simulink model "Project3_System_partA"  (R2018b)
settings: Solver=VariableStepAuto  StartTime=0.0  StopTime=10  FixedStep=.001  MaxStep=.001  RelTol=1e-6  EnableMultiTasking=on
values from neighbouring files (symbols this model uses):
  Kd = 700    [SimRun.m]
  Kp = 1000    [SimRun.m]
  n = link.inertia*(iwdot) + cross(iw, link.inertia*iw)    [newtonEuler.m]
  points = points3D    [SimRun.m]
  transPercent = 0.025    [SimRun.m]
(part 4 of 4)

== matlab function Project3_System_partA/MATLAB Function ==
  data: theta input; theta_ddot input; torque output; theta_dot input
function torque = newton_euler( theta, theta_ddot, theta_dot )
%#codegen
coder.extrinsic('evalin');
coder.extrinsic('newtonEuler');

persistent linkList boundry_conditions;

if isempty(linkList)
    linkList = evalin('base','linkList');
    boundry_conditions.base_angular_velocity = [0;0;0];
    boundry_conditions.base_angular_acceleration = [0;0;0];
    boundry_conditions.base_linear_acceleration = [0;0;9.8];
    boundry_conditions.distal_force = [0;0;0];
    boundry_conditions.distal_torque = [0;0;0];
end

theta(2) = theta(2)-pi/2; % put in DH frame
torque = zeros(6,1);
torque = newtonEuler(linkList,theta,theta_dot,theta_ddot,boundry_conditions);


end

== matlab function Project3_System_partA/ABB Arm Dynamics/Laser Tracking ==
  data: theta input; pose output
function pose = laserTracker(theta)
%#codegen
coder.extrinsic('evalin');
persistent Sim_Exact;

if isempty(Sim_Exact)
    Sim_Exact = evalin('base','Sim_Exact');
end


th1 = theta(1);
th2 = theta(2);
th3 = theta(3);
th4 = theta(4);
th5 = theta(5);
th6 = theta(6);


if(Sim_Exact)
    pose = [ sin(th6)*(cos(th4)*sin(th1) + sin(th4)*(cos(th1)*sin(th2)*sin(th3) - cos(th1)*cos(th2)*cos(th3))) + cos(th6)*(cos(th5)*(sin(th1)*sin(th4) - cos(th4)*(cos(th1)*sin(th2)*sin(th3) - cos(th1)*cos(th2)*cos(th3))) - sin(th5)*(cos(th1)*cos(th2)*sin(th3) + cos(th1)*cos(th3)*sin(th2))), cos(th6)*(cos(th4)*sin(th1) + sin(th4)*(cos(th1)*sin(th2)*sin(th3) - cos(th1)*cos(th2)*cos(th3))) - sin(th6)*(cos(th5)*(sin(th1)*sin(th4) - cos(th4)*(cos(th1)*sin(th2)*sin(th3) - cos(th1)*cos(th2)*cos(th3))) - sin(th5)*(cos(th1)*cos(th2)*sin(th3) + cos(th1)*cos(th3)*sin(th2))), - sin(th5)*(sin(th1)*sin(th4) - cos(th4)*(cos(th1)*sin(th2)*sin(th3) - cos(th1)*cos(th2)*cos(th3))) - cos(th5)*(cos(th1)*cos(th2)*sin(th3) + cos(th1)*cos(th3)*sin(th2)), (27*cos(th1)*cos(th2))/100 - (9*sin(th5)*(sin(th1)*sin(th4) - cos(th4)*(cos(th1)*sin(th2)*sin(th3) - cos(th1)*cos(th2)*cos(th3))))/125 - (9*cos(th5)*(cos(th1)*cos(th2)*sin(th3) + cos(th1)*cos(th3)*sin(th2)))/125 - (7*cos(th1)*sin(th2)*sin(th3))/100 + (7*cos(th1)*cos(th2)*cos(th3))/100 - (151*cos(th1)*cos(th2)*sin(th3))/500 - (151*cos(th1)*cos(th3)*sin(th2))/500;
        - sin(th6)*(cos(th1)*cos(th4) - sin(th4)*(sin(th1)*sin(th2)*sin(th3) - cos(th2)*cos(th3)*sin(th1))) - cos(th6)*(cos(th5)*(cos(th1)*sin(th4) + cos(th4)*(sin(th1)*sin(th2)*sin(th3) - cos(th2)*cos(th3)*sin(th1))) + sin(th5)*(cos(th2)*sin(th1)*sin(th3) + cos(th3)*sin(th1)*sin(th2))), sin(th6)*(cos(th5)*(cos(th1)*sin(th4) + cos(th4)*(sin(th1)*sin(th2)*sin(th3) - cos(th2)*cos(th3)*sin(th1))) + sin(th5)*(cos(th2)*sin(th1)*sin(th3) + cos(th3)*sin(th1)*sin(th2))) - cos(th6)*(cos(th1)*cos(th4) - sin(th4)*(sin(th1)*sin(th2)*sin(th3) - cos(th2)*cos(th3)*sin(th1))), sin(th5)*(cos(th1)*sin(th4) + cos(th4)*(sin(th1)*sin(th2)*sin(th3) - cos(th2)*cos(th3)*sin(th1))) - cos(th5)*(cos(th2)*sin(th1)*sin(th3) + cos(th3)*sin(th1)*sin(th2)), (27*cos(th2)*sin(th1))/100 + (9*sin(th5)*(cos(th1)*sin(th4) + cos(th4)*(sin(th1)*sin(th2)*sin(th3) - cos(th2)*cos(th3)*sin(th1))))/125 - (9*cos(th5)*(cos(th2)*sin(th1)*sin(th3) + cos(th3)*sin(th1)*sin(th2)))/125 - (151*cos(th2)*sin(th1)*sin(th3))/500 - (151*cos(th3)*sin(th1)*sin(th2))/500 - (7*sin(th1)*sin(th2)*sin(th3))/100 + (7*cos(th2)*cos(th3)*sin(th1))/100;
        sin(th4)*sin(th6)*(cos(th2)*sin(th3) + cos(th3)*sin(th2)) - cos(th6)*(sin(th5)*(cos(th2)*cos(th3) - sin(th2)*sin(th3)) + cos(th4)*cos(th5)*(cos(th2)*sin(th3) + cos(th3)*sin(th2))), sin(th6)*(sin(th5)*(cos(th2)*cos(th3) - sin(th2)*sin(th3)) + cos(th4)*cos(th5)*(cos(th2)*sin(th3) + cos(th3)*sin(th2))) + cos(th6)*sin(th4)*(cos(th2)*sin(th3) + cos(th3)*sin(th2)), cos(th4)*sin(th5)*(cos(th2)*sin(th3) + cos(th3)*sin(th2)) - cos(th5)*(cos(th2)*cos(th3) - sin(th2)*sin(th3)), (151*sin(th2)*sin(th3))/500 - (151*cos(th2)*cos(th3))/500 - (7*cos(th2)*sin(th3))/100 - (7*cos(th3)*sin(th2))/100 - (27*sin(th2))/100 - (9*cos(th5)*(cos(th2)*cos(th3) - sin(th2)*sin(th3)))/125 + (9*cos(th4)*sin(th5)*(cos(th2)*sin(th3) + cos(th3)*sin(th2)))/125 + 29/100;
        0, 0, 0, 1];
else
    
    pose = [ sin(th6)*(cos(th4)*sin(th1) + sin(th4)*(cos(th1)*sin(th2)*sin(th3) - cos(th1)*cos(th2)*cos(th3))) + cos(th6)*(cos(th5)*(sin(th1)*sin(th4) - cos(th4)*(cos(th1)*sin(th2)*sin(th3) - cos(th1)*cos(th2)*cos(th3))) - sin(th5)*(cos(th1)*cos(th2)*sin(th3) + cos(th1)*cos(th3)*sin(th2))), cos(th6)*(cos(th4)*sin(th1) + sin(th4)*(cos(th1)*sin(th2)*sin(th3) - cos(th1)*cos(th2)*cos(th3))) - sin(th6)*(cos(th5)*(sin(th1)*sin(th4) - cos(th4)*(cos(th1)*sin(th2)*sin(th3) - cos(th1)*cos(th2)*cos(th3))) - sin(th5)*(cos(th1)*cos(th2)*sin(th3) + cos(th1)*cos(th3)*sin(th2))), - sin(th5)*(sin(th1)*sin(th4) - cos(th4)*(cos(th1)*sin(th2)*sin(th3) - cos(th1)*cos(th2)*cos(th3))) - cos(th5)*(cos(th1)*cos(th2)*sin(th3) + cos(th1)*cos(th3)*sin(th2)), (151838081588107*cos(th1)*cos(th2))/562949953421312 - (123928564092639*sin(th1))/72057594037927936 - (7184037743251309*cos(th1))/36893488147419103232 - (7330531551818703*cos(th4)*sin(th1))/36893488147419103232 - (5489399374888815*sin(th1)*sin(th4))/9223372036854775808 + (970893499285375*cos(th5)*(sin(th1)*sin(th4) - cos(th4)*(cos(th1)*sin(th2)*sin(th3) - cos(th1)*cos(th2)*cos(th3))))/9223372036854775808 - (5192391675427195*sin(th5)*(sin(th1)*sin(th4) - cos(th4)*(cos(th1)*sin(th2)*sin(th3) - cos(th1)*cos(th2)*cos(th3))))/72057594037927936 + (1663072680156839*sin(th6)*(cos(th4)*sin(th1) + sin(th4)*(cos(th1)*sin(th2)*sin(th3) - cos(th1)*cos(th2)*cos(th3))))/2305843009213693952 + (1663072680156839*cos(th6)*(cos(th5)*(sin(th1)*sin(th4) - cos(th4)*(cos(th1)*sin(th2)*sin(th3) - cos(th1)*cos(th2)*cos(th3))) - sin(th5)*(cos(th1)*cos(th2)*sin(th3) + cos(th1)*cos(th3)*sin(th2))))/2305843009213693952 + (5489399374888815*cos(th4)*(cos(th1)*sin(th2)*sin(th3) - cos(th1)*cos(th2)*cos(th3)))/9223372036854775808 - (5192391675427195*cos(th5)*(cos(th1)*cos(th2)*sin(th3) + cos(th1)*cos(th3)*sin(th2)))/72057594037927936 - (7330531551818703*sin(th4)*(cos(th1)*sin(th2)*sin(th3) - cos(th1)*cos(th2)*cos(th3)))/36893488147419103232 - (970893499285375*sin(th5)*(cos(th1)*cos(th2)*sin(th3) + cos(th1)*cos(th3)*sin(th2)))/9223372036854775808 - (1259578569946919*cos(th1)*sin(th2)*sin(th3))/18014398509481984 + (1259578569946919*cos(th1)*cos(th2)*cos(th3))/18014398509481984 - (5430591396830085*cos(th1)*cos(th2)*sin(th3))/18014398509481984 - (5430591396830085*cos(th1)*cos(th3)*sin(th2))/18014398509481984;
        - sin(th6)*(cos(th1)*cos(th4) - sin(th4)*(sin(th1)*sin(th2)*sin(th3) - cos(th2)*cos(th3)*sin(th1))) - cos(th6)*(cos(th5)*(cos(th1)*sin(th4) + cos(th4)*(sin(th1)*sin(th2)*sin(th3) - cos(th2)*cos(th3)*sin(th1))) + sin(th5)*(cos(th2)*sin(th1)*sin(th3) + cos(th3)*sin(th1)*sin(th2))), sin(th6)*(cos(th5)*(cos(th1)*sin(th4) + cos(th4)*(sin(th1)*sin(th2)*sin(th3) - cos(th2)*cos(th3)*sin(th1))) + sin(th5)*(cos(th2)*sin(th1)*sin(th3) + cos(th3)*sin(th1)*sin(th2))) - cos(th6)*(cos(th1)*cos(th4) - sin(th4)*(sin(th1)*sin(th2)*sin(th3) - cos(th2)*cos(th3)*sin(th1))), sin(th5)*(cos(th1)*sin(th4) + cos(th4)*(sin(th1)*sin(th2)*sin(th3) - cos(th2)*cos(th3)*sin(th1))) - cos(th5)*(cos(th2)*sin(th1)*sin(th3) + cos(th3)*sin(th1)*sin(th2)), (123928564092639*cos(th1))/72057594037927936 - (7184037743251309*sin(th1))/36893488147419103232 + (7330531551818703*cos(th1)*cos(th4))/36893488147419103232 + (151838081588107*cos(th2)*sin(th1))/562949953421312 + (5489399374888815*cos(th1)*sin(th4))/9223372036854775808 - (970893499285375*cos(th5)*(cos(th1)*sin(th4) + cos(th4)*(sin(th1)*sin(th2)*sin(th3) - cos(th2)*cos(th3)*sin(th1))))/9223372036854775808 + (5192391675427195*sin(th5)*(cos(th1)*sin(th4) + cos(th4)*(sin(th1)*sin(th2)*sin(th3) - cos(th2)*cos(th3)*sin(th1))))/72057594037927936 - (1663072680156839*sin(th6)*(cos(th1)*cos(th4) - sin(th4)*(sin(th1)*sin(th2)*sin(th3) - cos(th2)*cos(th3)*sin(th1))))/2305843009213693952 + (5489399374888815*cos(th4)*(sin(th1)*sin(th2)*sin(th3) - cos(th2)*cos(th3)*sin(th1)))/9223372036854775808 - (5192391675427195*cos(th5)*(cos(th2)*sin(th1)*sin(th3) + cos(th3)*sin(th1)*sin(th2)))/72057594037927936 - (1663072680156839*cos(th6)*(cos(th5)*(cos(th1)*sin(th4) + cos(th4)*(sin(th1)*sin(th2)*sin(th3) - cos(th2)*cos(th3)*sin(th1))) + sin(th5)*(cos(th2)*sin(th1)*sin(th3) + cos(th3)*sin(th1)*sin(th2))))/2305843009213693952 - (7330531551818703*sin(th4)*(sin(th1)*sin(th2)*sin(th3) - cos(th2)*cos(th3)*sin(th1)))/36893488147419103232 - (970893499285375*sin(th5)*(cos(th2)*sin(th1)*sin(th3) + cos(th3)*sin(th1)*sin(th2)))/9223372036854775808 - (5430591396830085*cos(th2)*sin(th1)*sin(th3))/18014398509481984 - (5430591396830085*cos(th3)*sin(th1)*sin(th2))/18014398509481984 - (1259578569946919*sin(th1)*sin(th2)*sin(th3))/18014398509481984 + (1259578569946919*cos(th2)*cos(th3)*sin(th1))/18014398509481984;
        sin(th4)*sin(th6)*(cos(th2)*sin(th3) + cos(th3)*sin(th2)) - cos(th6)*(sin(th5)*(cos(th2)*cos(th3) - sin(th2)*sin(th3)) + cos(th4)*cos(th5)*(cos(th2)*sin(th3) + cos(th3)*sin(th2))), sin(th6)*(sin(th5)*(cos(th2)*cos(th3) - sin(th2)*sin(th3)) + cos(th4)*cos(th5)*(cos(th2)*sin(th3) + cos(th3)*sin(th2))) + cos(th6)*sin(th4)*(cos(th2)*sin(th3) + cos(th3)*sin(th2)), cos(th4)*sin(th5)*(cos(th2)*sin(th3) + cos(th3)*sin(th2)) - cos(th5)*(cos(th2)*cos(th3) - sin(th2)*sin(th3)), (5430591396830085*sin(th2)*sin(th3))/18014398509481984 - (5430591396830085*cos(th2)*cos(th3))/18014398509481984 - (1259578569946919*cos(th2)*sin(th3))/18014398509481984 - (1259578569946919*cos(th3)*sin(th2))/18014398509481984 - (1663072680156839*cos(th6)*(sin(th5)*(cos(th2)*cos(th3) - sin(th2)*sin(th3)) + cos(th4)*cos(th5)*(cos(th2)*sin(th3) + cos(th3)*sin(th2))))/2305843009213693952 - (151838081588107*sin(th2))/562949953421312 + (5489399374888815*cos(th4)*(cos(th2)*sin(th3) + cos(th3)*sin(th2)))/9223372036854775808 - (5192391675427195*cos(th5)*(cos(th2)*cos(th3) - sin(th2)*sin(th3)))/72057594037927936 - (7330531551818703*sin(th4)*(cos(th2)*sin(th3) + cos(th3)*sin(th2)))/36893488147419103232 - (970893499285375*sin(th5)*(cos(th2)*cos(th3) - sin(th2)*sin(th3)))/9223372036854775808 - (970893499285375*cos(th4)*cos(th5)*(cos(th2)*sin(th3) + cos(th3)*sin(th2)))/9223372036854775808 + (5192391675427195*cos(th4)*sin(th5)*(cos(th2)*sin(th3) + cos(th3)*sin(th2)))/72057594037927936 + (1663072680156839*sin(th4)*sin(th6)*(cos(th2)*sin(th3) + cos(th3)*sin(th2)))/2305843009213693952 + 325695105792877/1125899906842624;
        0, 0, 0, 1];
end

== matlab function Project3_System_partA/MATLAB Function1 ==
  data: t input; theta_des output; points input; n input
function theta_des = abb(t,points,n)
theta_des = zeros(length(t),7);
thetaa = zeros(length(t),7);
th_last=[0;-pi/2;0;0;0;0];
th1=0;
th2=0;
th3=0;
th4=0;
th5=0;
th6=0;
R=zeros(3,3);
x_vec=zeros(3,1);
y_vec=zeros(3,1);
z_vec=zeros(3,1);
% [n,V,p] = affine_fit(points);
z_vec=real(n);

thetaa(1,2:7)=-1*th_last';
thetaa(1,1)=t(1);
diff=points(2,:)-points(1,:);
x_vec=diff'/norm(diff);
y_vec=cpMap(z_vec)*x_vec;
R=[x_vec y_vec z_vec];
[th1,th2,th3,th4,th5,th6,~]=abbInvKine([R points(1,:)';0 0 0 1],th_last);
thetaa(2,2:7)=[th1,th2,th3,th4,th5,th6];
thetaa(2,1)=t(2);
[th1,th2,th3,th4,th5,th6,~]=abbInvKine([R points(1,:)';0 0 0 1],th_last);
thetaa(3,2:7)=[th1,th2,th3,th4,th5,th6];
thetaa(3,1)=t(3);
for i=3:length(t)-2
    diff=points(i-1,:)-points(i-2,:);
    x_vec=diff'/norm(diff);
    y_vec=cpMap(z_vec)*x_vec;
    R=[x_vec y_vec z_vec];
[th1,th2,th3,th4,th5,th6,~]=abbInvKine([R points(i-1,:)';0 0 0 1],thetaa(i,2:7)');
thetaa(i+1,2:7)=[th1,th2,th3,th4,th5,th6];
% for j=2:7
% if thetaa(i+1,j)*thetaa(i,j)' <0
% thetaa(i+1,j)=-1*thetaa(i+1,j);
% end
% end
thetaa(i+1,1)=t(i+1);
thetaa(i+2,2:7)=thetaa(i+1,2:7);
thetaa(i+2,1)=t(i+2);
end
theta_des = thetaa;
end

== matlab function Project3_System_partA/MATLAB Function2 ==
  data: t input double; theta output double; trajectory input double; transPercent input double; theta_dot output double
function [theta,theta_dot] = constAccelInterp(t,trajectory,transPercent)
pTime = trajectory(:,1);
[n,m] = size(trajectory);
thetaa = zeros(1,m-1);
thetaa_dot = zeros(1,m-1);
a = zeros(1,m-1);
for j = 2:n-1
    if j-1==1 && t>=pTime(j-1,1) && t<=(pTime(j-1,1)+transPercent)
        for i = 2:m
            thetaa(1,i-1) = trajectory(j-1,i) +...
                (((trajectory(j,i)-trajectory(j-1,i))*((t-pTime(j-1,1)+transPercent)^2))/(4*transPercent*(pTime(j,1)-pTime(j-1,1))));
            thetaa_dot(1,i-1) = (((trajectory(j,i)-trajectory(j-1,i))*(t-pTime(j-1,1)+transPercent))/(2*transPercent*(pTime(j,1)-pTime(j-1,1))));
            a(1,i-1) = ((trajectory(j,i)-trajectory(j-1,i))/(2*transPercent*(pTime(j,1)-pTime(j-1,1))));
        end
        break;
    elseif j+1==n && t>=(pTime(j+1,1)-transPercent) && t<=pTime(j+1,1)
        for i = 2:m
            thetaa(1,i-1) = trajectory(j+1,i) - ...
                (((trajectory(j+1,i)-trajectory(j,i))*((t-pTime(j+1,1)-transPercent)^2))/(4*transPercent*(pTime(j+1,1)-pTime(j,1))));
            thetaa_dot(1,i-1) = -(((trajectory(j+1,i)-trajectory(j,i))*(t-pTime(j+1,1)-transPercent))/(2*transPercent*(pTime(j+1,1)-pTime(j,1))));
            a(1,i-1) = -((trajectory(j+1,i)-trajectory(j,i))/(2*transPercent*(pTime(j+1,1)-pTime(j,1))));
        end
        break;
    elseif t>=(pTime(j-1,1)+transPercent) && t<=(pTime(j,1)-transPercent)
        for i = 2:m
            thetaa(1,i-1) = trajectory(j,i)-(((pTime(j,1)-t)*(trajectory(j,i)-...
                trajectory(j-1,i)))/(pTime(j,1)-pTime(j-1,1)));
            thetaa_dot(1,i-1) = (trajectory(j,i)-trajectory(j-1,i))/(pTime(j,1)-pTime(j-1,1));
            a(1,i-1) = 0.0;
        end
        break;
    elseif t>=(pTime(j,1)-transPercent) && t<=(pTime(j,1)+transPercent)
        for i = 2:m
            thetaa(1,i-1) = trajectory(j,i) - ...
                (((trajectory(j,i)-trajectory(j-1,i))*((t-pTime(j,1)-transPercent)^2))/(4*transPercent*(pTime(j,1)-pTime(j-1,1)))) +...
                (((trajectory(j+1,i)-trajectory(j,i))*((t-pTime(j,1)+transPercent)^2))/(4*transPercent*(pTime(j+1,1)-pTime(j,1))));
            thetaa_dot(1,i-1) = -(((trajectory(j,i)-trajectory(j-1,i))*(t-pTime(j,1)-transPercent))/(2*transPercent*(pTime(j,1)-pTime(j-1,1)))) +...
                (((trajectory(j+1,i)-trajectory(j,i))*(t-pTime(j,1)+transPercent))/(2*transPercent*(pTime(j+1,1)-pTime(j,1))));
            a(1,i-1) = -((trajectory(j,i)-trajectory(j-1,i))/(2*transPercent*(pTime(j,1)-pTime(j-1,1)))) + ...
                ((trajectory(j+1,i)-trajectory(j,i))/(2*transPercent*(pTime(j+1,1)-pTime(j,1))));
        end
        break;
    elseif t>=(pTime(j,1)+transPercent) && t<=(pTime(j+1,1)-transPercent)
        for i = 2:m
            thetaa(1,i-1) = trajectory(j,i)+(((t-pTime(j,1))*(trajectory(j+1,i)-...
                trajectory(j,i)))/(pTime(j+1,1)-pTime(j,1)));
            thetaa_dot(1,i-1) = (trajectory(j+1,i)-trajectory(j,i))/(pTime(j+1,1)-pTime(j,1));
            a(1,i-1) = 0.0;
        end
        break;
    end
end
theta=thetaa;
theta_dot=thetaa_dot;
end

== matlab function Project3_System_partA/MATLAB Function9 ==
  data: theta input; X output
function X = fwdKine(theta)
d1 = 0.29;
a2 = 0.270;
a3 = 0.070;
d4 = 0.302;
d6 = 0.072;

rcom1 = [0;-d1/2;0];
rcom2 = [-a2/2;0;0];
rcom3 = [-a3/2;0;0];
rcom4 = [0;-d4/2;0];
rcom5 = [0;0;0];
rcom6 = [0; -d6/2;0];

rad1 = .2/2; h1 = d1;   m1 = 8050*h1*rad1^2*pi;
rad2 = .15/2; h2 = a2;   m2 = 8050*h2*rad2^2*pi;
rad3 = .1/2; h3 = a3;  m3 = 8050*h3*rad3^2*pi;
rad4 = .1/2; h4 = d4;  m4 = 8050*h4*rad4^2*pi;
rad5 = .05/2; h5 = .125; m5 = 8050*h5*rad5^2*pi;
rad6 = .05/2; h6 = d6;  m6 = 8050*h6*rad6^2*pi;

J1 = diag(m1*[1/12*(3*rad1^2+h1^2),rad1^2/2,1/12*(3*rad1^2+h1^2)]);
J2 = diag(m2*[rad2^2/2,1/12*(3*rad2^2+h2^2),1/12*(3*rad2^2+h2^2)]);
J3 = diag(m3*[rad3^2/2,1/12*(3*rad3^2+h3^2),1/12*(3*rad3^2+h3^2)]);
J4 = diag(m4*[1/12*(3*rad4^2+h4^2),rad4^2/2,1/12*(3*rad4^2+h4^2)]);
J5 = diag(m5*[1/12*(3*rad5^2+h5^2),rad5^2/2,1/12*(3*rad5^2+h5^2)]);
J6 = diag(m6*[1/12*(3*rad6^2+h6^2),rad6^2/2,1/12*(3*rad6^2+h6^2)]);

L1 = createLink(0,d1,-pi/2,[],rcom1, m1,J1);
L2 = createLink(a2,0,0,[],rcom2, m2,J2);
L3 = createLink(a3,0,-pi/2,[],rcom3, m3,J3);
L4 = createLink(0,d4,pi/2,[],rcom4, m4,J4);
L5 = createLink(0,0,-pi/2,[],rcom5, m5,J5);
L6 = createLink(0,d6,0,[],rcom6, m6,J6);

linkList = [L1;L2;L3;L4;L5;L6]';

X1=zeros(3,1);
k=zeros(3,1);
omega=zeros(3,1);
Y=zeros(4,4);

Y=dhFwdKine(linkList,theta);
% R=Y(1:3,1:3);
% [k, theta1] = rot2AngleAxis(R);
% omega=theta1*k;
X=Y(1:3,4);
% X=[X1;omega];
end
